simulink model "im_model_test1"  (R2022b)
settings: Solver=VariableStepAuto  StartTime=0.0  StopTime=0.5  MaxStep=0.0005  RelTol=1e-3
values from neighbouring files (symbols this model uses):
  B = 0.00825    [im_params.m]
  J = 0.033    [im_params.m]
  K1 = (-Rs*Lr^2-Rr*Lm^2)/(Lr*w)    (= -230.46612657)    [im_params.m]
  K2 = (Rr*Lm)/(Lr*w)    (= 1155.33638605)    [im_params.m]
  K3 = Lm/w    (= 163.672654691)    [im_params.m]
  K4 = Lr/w    (= 169.660678643)    [im_params.m]
  K5 = Rr*Lm/Lr    (= 0.578823529412)    [im_params.m]
  K6 = -Rr/Lr    (= -7.05882352941)    [im_params.m]
  Lm = 0.082    [im_params.m]
  Lr = 0.085    [im_params.m]
  pole = 4    [im_params.m]
settings Model: Creator=jack  LastModifiedBy=jack

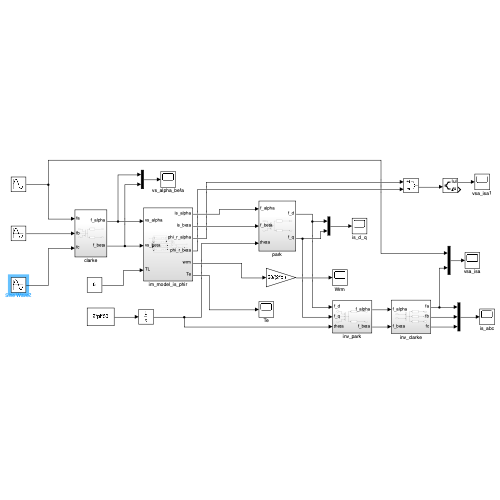
[thumbnail: Simulink's stored preview of the top-level diagram]
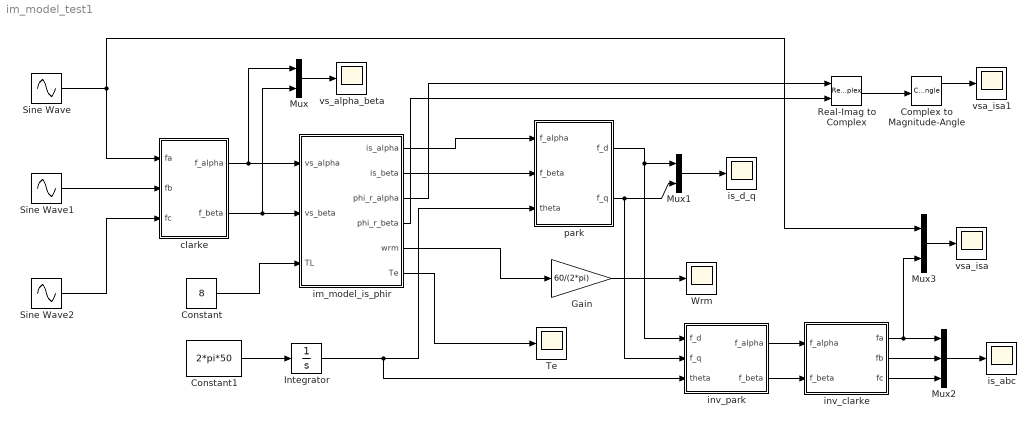
== system im_model_test1 ==
  Complex to Magnitude-Angle : ComplexToMagnitudeAngle
  Constant : Constant  Value=8
  Constant1 : Constant  Value=2*pi*50
  Gain : Gain  Gain=60/(2*pi)
  Integrator : Integrator
  Mux : Mux  Inputs=2
  Mux1 : Mux  Inputs=2
  Mux2 : Mux  Inputs=3
  Mux3 : Mux  Inputs=2
  Real-Imag to Complex : RealImagToComplex
  Sine Wave : Sin  Amplitude=220*1.414  Frequency=2*pi*50  SampleTime=0
  Sine Wave1 : Sin  Amplitude=220*1.414  Frequency=2*pi*50  Phase=-2*pi/3  SampleTime=0
  Sine Wave2 : Sin  Amplitude=220*1.414  Frequency=2*pi*50  Phase=-4*pi/3  SampleTime=0
  Te : Scope
  Wrm : Scope
  clarke : Subsystem
  im_model_is_phir : Subsystem
  inv_clarke : Subsystem
  inv_park : Subsystem
  is_abc : Scope
  is_d_q : Scope
  park : Subsystem
  vs_alpha_beta : Scope
  vsa_isa : Scope
  vsa_isa1 : Scope
  wires:
  Sine Wave/1 -> clarke/1(fa), Mux3/1
  Sine Wave1/1 -> clarke/2(fb)
  Sine Wave2/1 -> clarke/3(fc)
  clarke/1(f_alpha) -> Mux/1, im_model_is_phir/1(vs_alpha)
  clarke/2(f_beta) -> Mux/2, im_model_is_phir/2(vs_beta)
  Constant/1 -> im_model_is_phir/3(TL)
  im_model_is_phir/1(is_alpha) -> park/1(f_alpha)
  im_model_is_phir/2(is_beta) -> park/2(f_beta)
  Constant1/1 -> Integrator/1
  Integrator/1 -> inv_park/3(theta), park/3(theta)
  im_model_is_phir/6(Te) -> Te/1
  Mux/1 -> vs_alpha_beta/1
  park/1(f_d) -> inv_park/1(f_d), Mux1/1
  park/2(f_q) -> inv_park/2(f_q), Mux1/2
  Mux1/1 -> is_d_q/1
  im_model_is_phir/5(wrm) -> Gain/1
  Gain/1 -> Wrm/1
  inv_park/1(f_alpha) -> inv_clarke/1(f_alpha)
  inv_park/2(f_beta) -> inv_clarke/2(f_beta)
  inv_clarke/1(fa) -> Mux3/2, Mux2/1
  inv_clarke/2(fb) -> Mux2/2
  inv_clarke/3(fc) -> Mux2/3
  Mux2/1 -> is_abc/1
  Mux3/1 -> vsa_isa/1
  im_model_is_phir/3(phi_r_alpha) -> Real-Imag to Complex/1
  im_model_is_phir/4(phi_r_beta) -> Real-Imag to Complex/2
  Real-Imag to Complex/1 -> Complex to Magnitude-Angle/1
  Complex to Magnitude-Angle/1 -> vsa_isa1/1

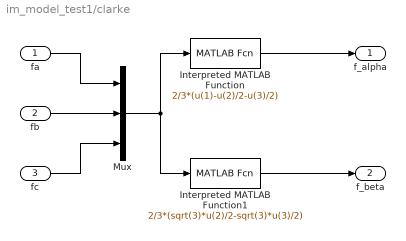
== system im_model_test1/clarke ==
  fa : Inport
  fb : Inport  Port=2
  fc : Inport  Port=3
  Interpreted MATLAB Function : MATLABFcn  MATLABFcn=2/3*(u(1)-u(2)/2-u(3)/2)
  Interpreted MATLAB Function1 : MATLABFcn  MATLABFcn=2/3*(sqrt(3)*u(2)/2-sqrt(3)*u(3)/2)
  Mux : Mux  Inputs=3
  f_alpha : Outport
  f_beta : Outport  Port=2
  wires:
  Interpreted MATLAB Function/1 -> f_alpha/1
  fa/1 -> Mux/1
  Mux/1 -> Interpreted MATLAB Function1/1, Interpreted MATLAB Function/1
  Interpreted MATLAB Function1/1 -> f_beta/1
  fc/1 -> Mux/3
  fb/1 -> Mux/2

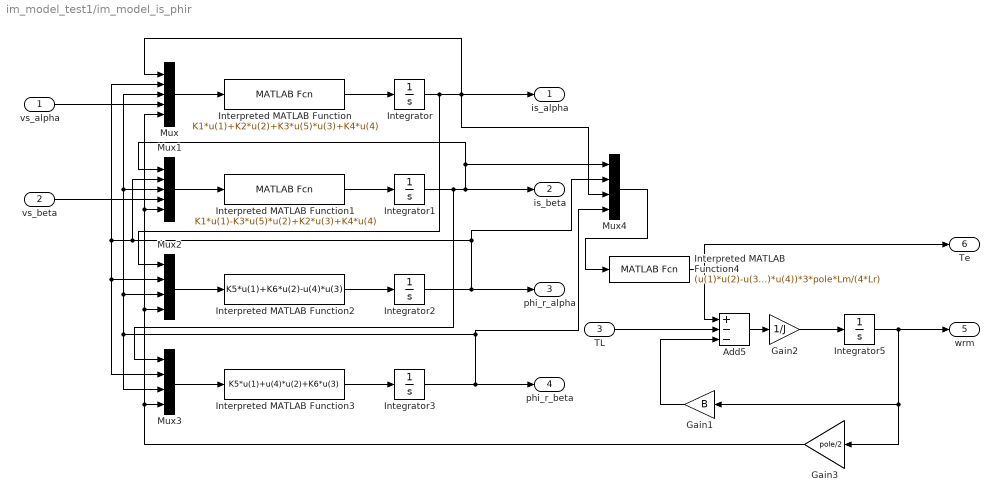
== system im_model_test1/im_model_is_phir ==
  vs_alpha : Inport
  vs_beta : Inport  Port=2
  TL : Inport  Port=3
  Add5 : Sum  Inputs=+--
  Gain1 : Gain  Gain=B
  Gain2 : Gain  Gain=1/J
  Gain3 : Gain  Gain=pole/2
  Integrator{,1..3,5} (5 alike) : Integrator
  Interpreted MATLAB Function : MATLABFcn  MATLABFcn=K1*u(1)+K2*u(2)+K3*u(5)*u(3)+K4*u(4)
  Interpreted MATLAB Function1 : MATLABFcn  MATLABFcn=K1*u(1)-K3*u(5)*u(2)+K2*u(3)+K4*u(4)
  Interpreted MATLAB Function2 : MATLABFcn  MATLABFcn=K5*u(1)+K6*u(2)-u(4)*u(3)
  Interpreted MATLAB Function3 : MATLABFcn  MATLABFcn=K5*u(1)+u(4)*u(2)+K6*u(3)
  Interpreted MATLAB Function4 : MATLABFcn  MATLABFcn=(u(1)*u(2)-u(3)*u(4))*3*pole*Lm/(4*Lr)
  Mux : Mux  Inputs=5
  Mux1 : Mux  Inputs=5
  Mux2 : Mux
  Mux3 : Mux
  Mux4 : Mux
  is_alpha : Outport
  is_beta : Outport  Port=2
  phi_r_alpha : Outport  Port=3
  phi_r_beta : Outport  Port=4
  wrm : Outport  Port=5
  Te : Outport  Port=6
  wires:
  Add5/1 -> Gain2/1
  Interpreted MATLAB Function2/1 -> Integrator2/1
  vs_beta/1 -> Mux1/4
  vs_alpha/1 -> Mux/4
  Mux3/1 -> Interpreted MATLAB Function3/1
  Interpreted MATLAB Function1/1 -> Integrator1/1
  Mux4/1 -> Interpreted MATLAB Function4/1
  Integrator1/1 -> Mux3/1, is_beta/1, Mux1/1, Mux4/1
  Gain1/1 -> Add5/3
  TL/1 -> Add5/2
  Interpreted MATLAB Function4/1 -> Te/1, Add5/1
  Integrator5/1 -> wrm/1, Gain1/1, Gain3/1
  Integrator2/1 -> phi_r_alpha/1, Mux4/2, Mux1/2, Mux/2, Mux3/2, Mux2/2
  Integrator3/1 -> phi_r_beta/1, Mux4/4, Mux3/3, Mux2/3, Mux/3, Mux1/3
  Mux1/1 -> Interpreted MATLAB Function1/1
  Interpreted MATLAB Function3/1 -> Integrator3/1
  Mux2/1 -> Interpreted MATLAB Function2/1
  Mux/1 -> Interpreted MATLAB Function/1
  Gain2/1 -> Integrator5/1
  Interpreted MATLAB Function/1 -> Integrator/1
  Integrator/1 -> Mux2/1, is_alpha/1, Mux4/3, Mux/1
  Gain3/1 -> Mux3/4, Mux2/4, Mux1/5, Mux/5

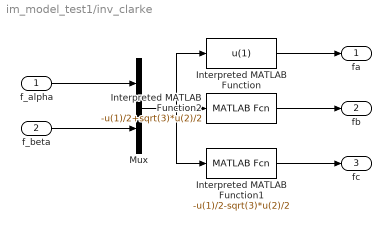
== system im_model_test1/inv_clarke ==
  f_alpha : Inport
  f_beta : Inport  Port=2
  Interpreted MATLAB Function : MATLABFcn  MATLABFcn=u(1)
  Interpreted MATLAB Function1 : MATLABFcn  MATLABFcn=-u(1)/2-sqrt(3)*u(2)/2
  Interpreted MATLAB Function2 : MATLABFcn  MATLABFcn=-u(1)/2+sqrt(3)*u(2)/2
  Mux : Mux  Inputs=2
  fa : Outport
  fb : Outport  Port=2
  fc : Outport  Port=3
  wires:
  Mux/1 -> Interpreted MATLAB Function/1, Interpreted MATLAB Function2/1, Interpreted MATLAB Function1/1
  f_alpha/1 -> Mux/1
  f_beta/1 -> Mux/2
  Interpreted MATLAB Function/1 -> fa/1
  Interpreted MATLAB Function2/1 -> fb/1
  Interpreted MATLAB Function1/1 -> fc/1

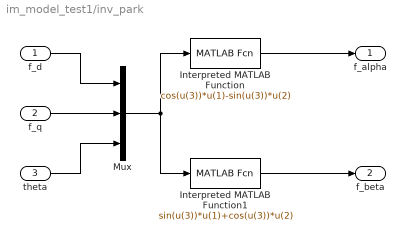
== system im_model_test1/inv_park ==
  f_d : Inport
  f_q : Inport  Port=2
  theta : Inport  Port=3
  Interpreted MATLAB Function : MATLABFcn  MATLABFcn=cos(u(3))*u(1)-sin(u(3))*u(2)
  Interpreted MATLAB Function1 : MATLABFcn  MATLABFcn=sin(u(3))*u(1)+cos(u(3))*u(2)
  Mux : Mux  Inputs=3
  f_alpha : Outport
  f_beta : Outport  Port=2
  wires:
  Interpreted MATLAB Function/1 -> f_alpha/1
  f_d/1 -> Mux/1
  Mux/1 -> Interpreted MATLAB Function1/1, Interpreted MATLAB Function/1
  Interpreted MATLAB Function1/1 -> f_beta/1
  theta/1 -> Mux/3
  f_q/1 -> Mux/2

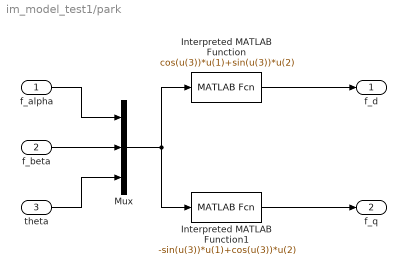
== system im_model_test1/park ==
  f_alpha : Inport
  f_beta : Inport  Port=2
  theta : Inport  Port=3
  Interpreted MATLAB Function : MATLABFcn  MATLABFcn=cos(u(3))*u(1)+sin(u(3))*u(2)
  Interpreted MATLAB Function1 : MATLABFcn  MATLABFcn=-sin(u(3))*u(1)+cos(u(3))*u(2)
  Mux : Mux  Inputs=3
  f_d : Outport
  f_q : Outport  Port=2
  wires:
  Interpreted MATLAB Function/1 -> f_d/1
  f_alpha/1 -> Mux/1
  Mux/1 -> Interpreted MATLAB Function1/1, Interpreted MATLAB Function/1
  Interpreted MATLAB Function1/1 -> f_q/1
  theta/1 -> Mux/3
  f_beta/1 -> Mux/2
